simulink model "lineraryzacja"  (R2021b)
settings: Solver=ode45  StartTime=0.0  StopTime=100.0  RelTol=1e-10
values from neighbouring files (symbols this model uses):
  G = 9.81    [edda.m]
  K0 = 1    [edda.m]
  K1 = 1    [edda.m]
  O1 = 3.1    [edda.m]
  O3 = 0.24    [edda.m]
  O4 = 0.77    [edda.m]
settings Model: Creator=mbober  LastModifiedBy=mbober
settings SolverCC: AlgebraicLoopSolver=TrustRegion
settings DebuggingCC: SFMachineParentedDataDiag=warning

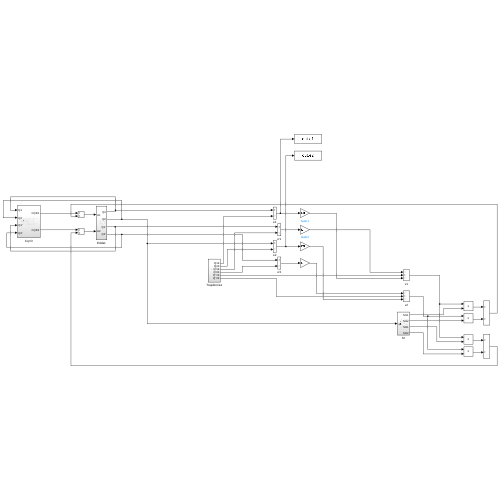
[thumbnail: Simulink's stored preview of the top-level diagram]
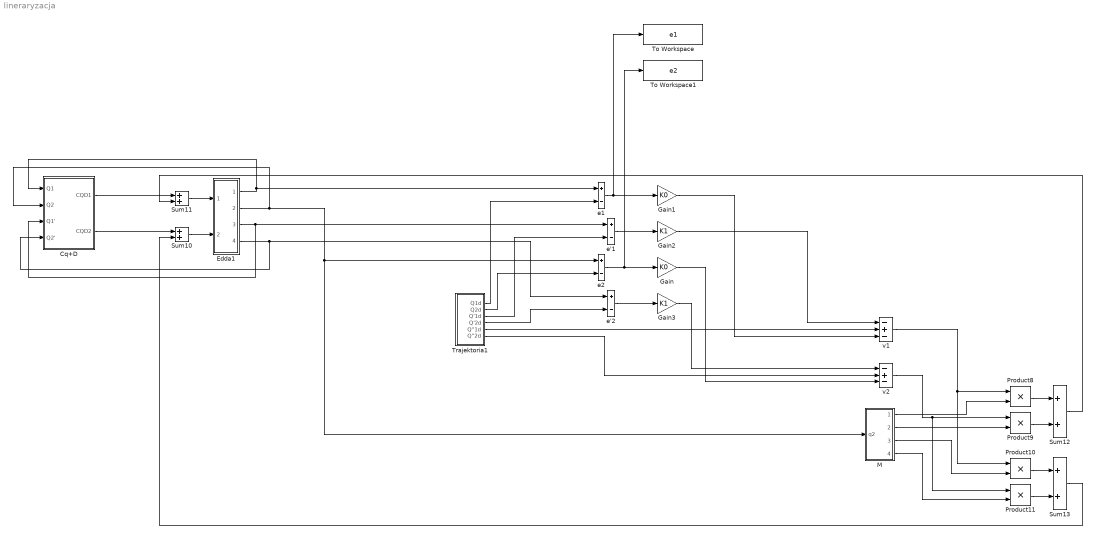
== system lineraryzacja ==
  Cq+D : Subsystem
  Edda1 : Subsystem
  Gain : Gain  Gain=K0
  Gain1 : Gain  Gain=K0
  Gain2 : Gain  Gain=K1
  Gain3 : Gain  Gain=K1
  M : Subsystem
  Product{8..11} (4 alike) : Product
  Sum{10..13} (4 alike) : Sum
  To Workspace : ToWorkspace  VariableName=e1  SampleTime=-1
  To Workspace1 : ToWorkspace  VariableName=e2  SampleTime=-1
  Trajektoria1 : Subsystem
  e'1 : Sum  Inputs=+-
  e'2 : Sum  Inputs=+-
  e1 : Sum  Inputs=+-
  e2 : Sum  Inputs=+-
  v1 : Sum  Inputs=-+-
  v2 : Sum  Inputs=-+-
  wires:
  e1/1 -> Gain1/1, To Workspace/1
  Edda1/1(Q1) -> Cq+D/1(Q1), e1/1
  Edda1/2(Q2) -> Cq+D/2(Q2), e2/1, M/1(q2)
  Sum10/1 -> Edda1/2(U2)
  Sum11/1 -> Edda1/1(U1)
  Trajektoria1/3(Q'1d) -> e'1/2
  Trajektoria1/1(Q1d) -> e1/2
  Trajektoria1/2(Q2d) -> e2/2
  Trajektoria1/4(Q'2d) -> e'2/2
  Trajektoria1/5(Q''1d) -> v1/2
  Trajektoria1/6(Q''2d) -> v2/2
  M/1(M11) -> Product8/2
  v1/1 -> Product10/1, Product8/1
  M/2(M12) -> Product9/2
  v2/1 -> Product11/1, Product9/1
  Product8/1 -> Sum12/1
  Product9/1 -> Sum12/2
  Sum12/1 -> Sum11/2
  Product10/1 -> Sum13/1
  Product11/1 -> Sum13/2
  M/3(M21) -> Product10/2
  M/4(M22) -> Product11/2
  Sum13/1 -> Sum10/2
  Cq+D/1(CQD1) -> Sum11/1
  Cq+D/2(CQD2) -> Sum10/1
  e2/1 -> Gain/1, To Workspace1/1
  Edda1/3(Q1') -> Cq+D/3(Q1'), e'1/1
  Edda1/4(Q2') -> Cq+D/4(Q2'), e'2/1
  Gain1/1 -> v1/3
  Gain/1 -> v2/3
  e'1/1 -> Gain2/1
  e'2/1 -> Gain3/1
  Gain2/1 -> v1/1
  Gain3/1 -> v2/1

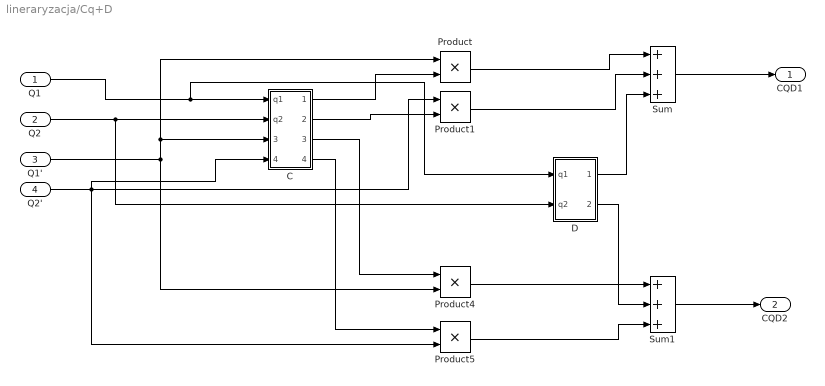
== system lineraryzacja/Cq+D ==
  Q1 : Inport
  Q2 : Inport  Port=2
  Q1' : Inport  Port=3
  Q2' : Inport  Port=4
  C : Subsystem
  D : Subsystem
  Product{,1,4..5} (4 alike) : Product
  Sum : Sum  Inputs=+++
  Sum1 : Sum  Inputs=+++
  CQD1 : Outport
  CQD2 : Outport  Port=2
  wires:
  C/1(C11) -> Product/2
  Q1'/1 -> C/3(q1'), Product/1, Product4/2
  Product/1 -> Sum/1
  Product1/1 -> Sum/2
  C/2(C12) -> Product1/2
  Q2'/1 -> C/4(q2'), Product5/2, Product1/1
  D/1(Out1) -> Sum/3
  C/3(C21) -> Product4/1
  C/4(C22) -> Product5/1
  Product4/1 -> Sum1/1
  Product5/1 -> Sum1/3
  D/2(Out2) -> Sum1/2
  Sum/1 -> CQD1/1
  Sum1/1 -> CQD2/1
  Q1/1 -> D/1(q1), C/1(q1)
  Q2/1 -> D/2(q2), C/2(q2)

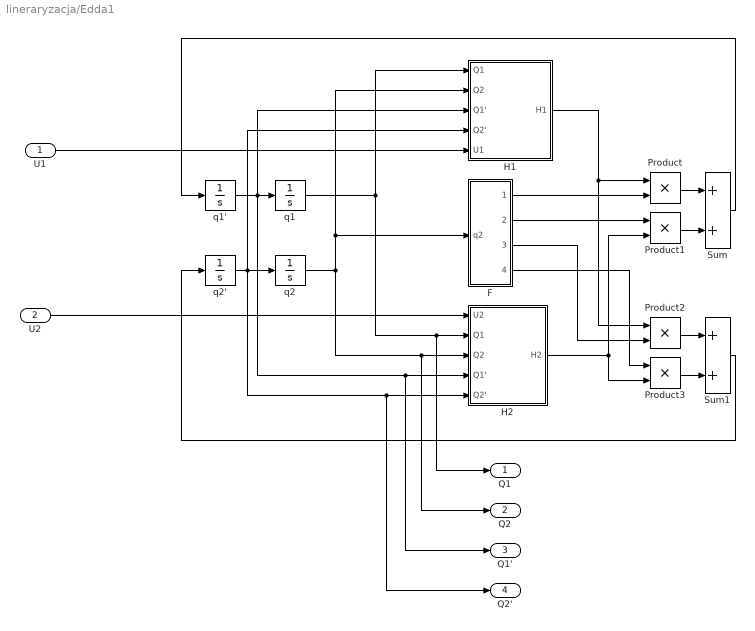
== system lineraryzacja/Edda1 ==
  U1 : Inport
  U2 : Inport  Port=2
  F : Subsystem
  H1 : Subsystem
  H2 : Subsystem
  Product{,1..3} (4 alike) : Product
  Sum : Sum
  Sum1 : Sum
  q1 : Integrator
  q1' : Integrator
  q2 : Integrator
  q2' : Integrator
  Q1 : Outport
  Q2 : Outport  Port=2
  Q1' : Outport  Port=3
  Q2' : Outport  Port=4
  wires:
  Product3/1 -> Sum1/2
  Product/1 -> Sum/1
  q2/1 -> F/1(q2), H1/2(Q2), Q2/1, H2/3(Q2)
  Sum1/1 -> q2'/1
  H1/1(H1) -> Product2/1, Product/1
  q2'/1 -> H1/4(Q2'), Q2'/1, H2/5(Q2'), q2/1
  Sum/1 -> q1'/1
  Product1/1 -> Sum/2
  F/3(F21) -> Product2/2
  H2/1(H2) -> Product3/2, Product1/2
  q1/1 -> H1/1(Q1), Q1/1, H2/2(Q1)
  Product2/1 -> Sum1/1
  F/1(F11) -> Product/2
  U1/1 -> H1/5(U1)
  F/2(F12) -> Product1/1
  q1'/1 -> H1/3(Q1'), Q1'/1, H2/4(Q1'), q1/1
  U2/1 -> H2/1(U2)
  F/4(F22) -> Product3/1

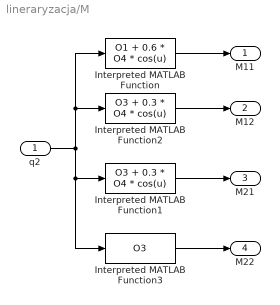
== system lineraryzacja/M ==
  q2 : Inport
  Interpreted MATLAB Function : MATLABFcn  MATLABFcn=O1 + 0.6 * O4 * cos(u)
  Interpreted MATLAB Function1 : MATLABFcn  MATLABFcn=O3 + 0.3 * O4 * cos(u)
  Interpreted MATLAB Function2 : MATLABFcn  MATLABFcn=O3 + 0.3 * O4 * cos(u)
  Interpreted MATLAB Function3 : MATLABFcn  MATLABFcn=O3
  M11 : Outport
  M12 : Outport  Port=2
  M21 : Outport  Port=3
  M22 : Outport  Port=4
  wires:
  Interpreted MATLAB Function3/1 -> M22/1
  Interpreted MATLAB Function/1 -> M11/1
  Interpreted MATLAB Function2/1 -> M12/1
  q2/1 -> Interpreted MATLAB Function/1, Interpreted MATLAB Function2/1, Interpreted MATLAB Function3/1, Interpreted MATLAB Function1/1
  Interpreted MATLAB Function1/1 -> M21/1

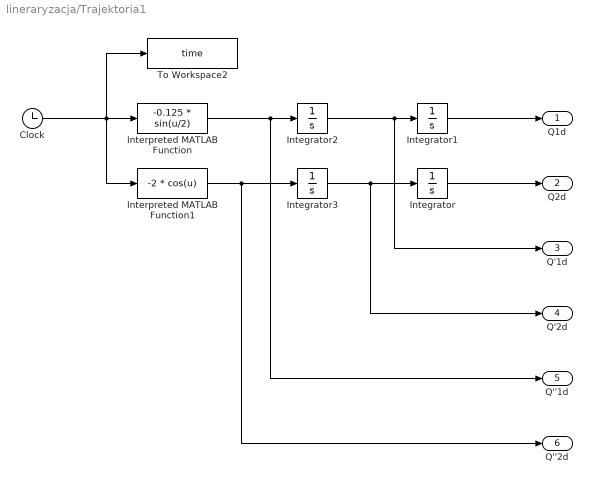
== system lineraryzacja/Trajektoria1 ==
  Clock : Clock
  Integrator : Integrator  InitialCondition=2
  Integrator1 : Integrator
  Integrator2 : Integrator  InitialCondition=0.25
  Integrator3 : Integrator
  Interpreted MATLAB Function : MATLABFcn  MATLABFcn=-0.125 * sin(u/2)
  Interpreted MATLAB Function1 : MATLABFcn  MATLABFcn=-2 * cos(u)
  To Workspace2 : ToWorkspace  VariableName=time  SampleTime=-1
  Q1d : Outport
  Q2d : Outport  Port=2
  Q'1d : Outport  Port=3
  Q'2d : Outport  Port=4
  Q''1d : Outport  Port=5
  Q''2d : Outport  Port=6
  wires:
  Integrator1/1 -> Q1d/1
  Interpreted MATLAB Function/1 -> Q''1d/1, Integrator2/1
  Integrator/1 -> Q2d/1
  Interpreted MATLAB Function1/1 -> Q''2d/1, Integrator3/1
  Clock/1 -> To Workspace2/1, Interpreted MATLAB Function1/1, Interpreted MATLAB Function/1
  Integrator2/1 -> Q'1d/1, Integrator1/1
  Integrator3/1 -> Q'2d/1, Integrator/1

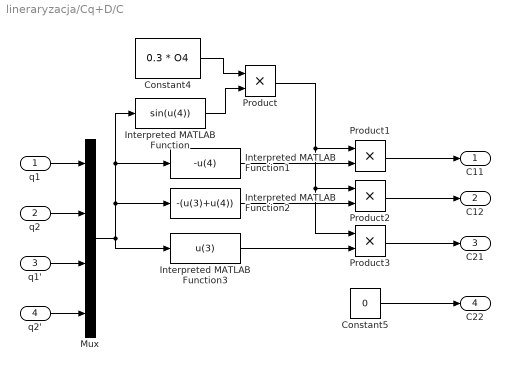
== system lineraryzacja/Cq+D/C ==
  q1 : Inport
  q2 : Inport  Port=2
  q1' : Inport  Port=3
  q2' : Inport  Port=4
  Constant4 : Constant  Value=0.3 * O4
  Constant5 : Constant  Value=0
  Interpreted MATLAB Function : MATLABFcn  MATLABFcn=sin(u(4))
  Interpreted MATLAB Function1 : MATLABFcn  MATLABFcn=-u(4)
  Interpreted MATLAB Function2 : MATLABFcn  MATLABFcn=-(u(3)+u(4))
  Interpreted MATLAB Function3 : MATLABFcn  MATLABFcn=u(3)
  Mux : Mux
  Product{,1..3} (4 alike) : Product
  C11 : Outport
  C12 : Outport  Port=2
  C21 : Outport  Port=3
  C22 : Outport  Port=4
  wires:
  Product3/1 -> C21/1
  Interpreted MATLAB Function1/1 -> Product1/2
  q2'/1 -> Mux/4
  Interpreted MATLAB Function2/1 -> Product2/2
  q2/1 -> Mux/2
  Constant4/1 -> Product/1
  Interpreted MATLAB Function/1 -> Product/2
  Product1/1 -> C11/1
  Interpreted MATLAB Function3/1 -> Product3/2
  q1'/1 -> Mux/3
  Mux/1 -> Interpreted MATLAB Function3/1, Interpreted MATLAB Function2/1, Interpreted MATLAB Function/1, Interpreted MATLAB Function1/1
  q1/1 -> Mux/1
  Constant5/1 -> C22/1
  Product/1 -> Product3/1, Product2/1, Product1/1
  Product2/1 -> C12/1

== system lineraryzacja/Cq+D/D ==
  q1 : Inport
  q2 : Inport  Port=2
  Interpreted MATLAB Function : MATLABFcn  MATLABFcn=(O1 * cos(u(2)) + O4 * cos(u(1)*u(2))) * G
  Interpreted MATLAB Function1 : MATLABFcn  MATLABFcn=O4 * cos(u(1)*u(2)) * G
  Mux : Mux  Inputs=2
  Out1 : Outport
  Out2 : Outport  Port=2
  wires:
  Interpreted MATLAB Function/1 -> Out1/1
  Interpreted MATLAB Function1/1 -> Out2/1
  Mux/1 -> Interpreted MATLAB Function1/1, Interpreted MATLAB Function/1
  q1/1 -> Mux/1
  q2/1 -> Mux/2

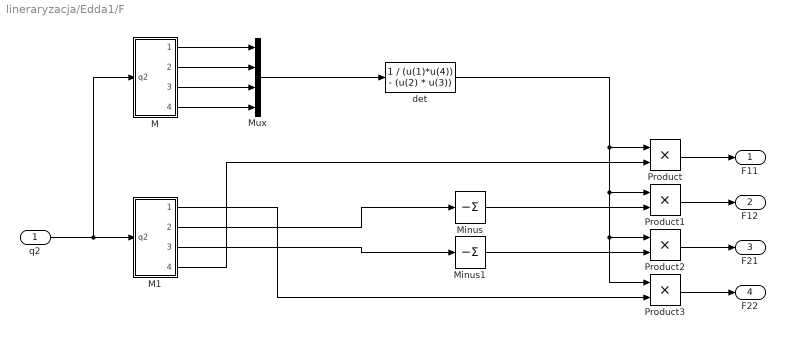
== system lineraryzacja/Edda1/F ==
  q2 : Inport
  M : Subsystem
  M1 : Subsystem
  Minus : Sum  Inputs=-
  Minus1 : Sum  Inputs=-
  Mux : Mux
  Product{,1..3} (4 alike) : Product
  det : MATLABFcn  MATLABFcn=1 / (u(1)*u(4)) - (u(2) * u(3))
  F11 : Outport
  F12 : Outport  Port=2
  F21 : Outport  Port=3
  F22 : Outport  Port=4
  wires:
  q2/1 -> M/1(q2), M1/1(q2)
  M1/2(M12) -> Minus/1
  M1/3(M21) -> Minus1/1
  Mux/1 -> det/1
  M/2(M12) -> Mux/2
  M/1(M11) -> Mux/1
  M/3(M21) -> Mux/3
  M/4(M22) -> Mux/4
  Product/1 -> F11/1
  Product1/1 -> F12/1
  Product2/1 -> F21/1
  Product3/1 -> F22/1
  det/1 -> Product3/1, Product2/1, Product1/1, Product/1
  M1/1(M11) -> Product3/2
  M1/4(M22) -> Product/2
  Minus/1 -> Product1/2
  Minus1/1 -> Product2/2

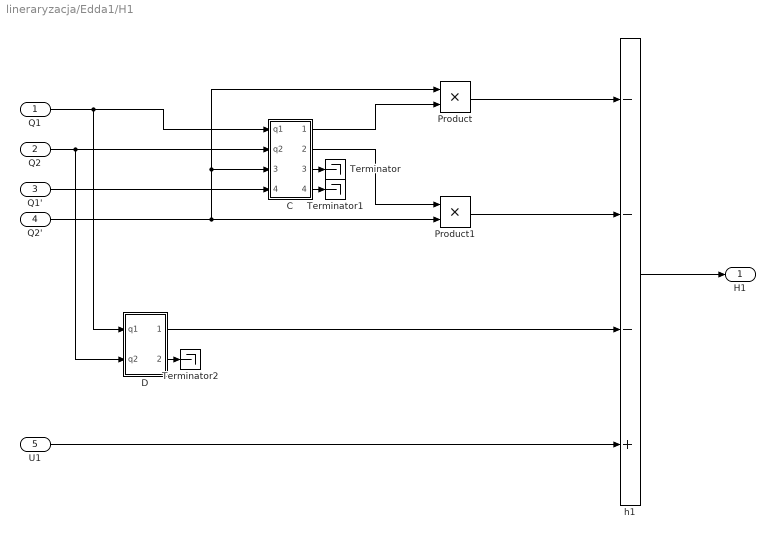
== system lineraryzacja/Edda1/H1 ==
  Q1 : Inport
  Q2 : Inport  Port=2
  Q1' : Inport  Port=3
  Q2' : Inport  Port=4
  U1 : Inport  Port=5
  C : Subsystem
  D : Subsystem
  Product : Product
  Product1 : Product
  Terminator : Terminator
  Terminator1 : Terminator
  Terminator2 : Terminator
  h1 : Sum  Inputs=---+
  H1 : Outport
  wires:
  U1/1 -> h1/4
  C/2(C12) -> Product1/1
  Product/1 -> h1/1
  Q1'/1 -> C/3(q1'), Product/1
  Product1/1 -> h1/2
  Q2/1 -> D/2(q2), C/2(q2)
  C/1(C11) -> Product/2
  Q1/1 -> D/1(q1), C/1(q1)
  D/1(Out1) -> h1/3
  Q2'/1 -> C/4(q2'), Product1/2
  h1/1 -> H1/1
  C/3(C21) -> Terminator/1
  C/4(C22) -> Terminator1/1
  D/2(Out2) -> Terminator2/1

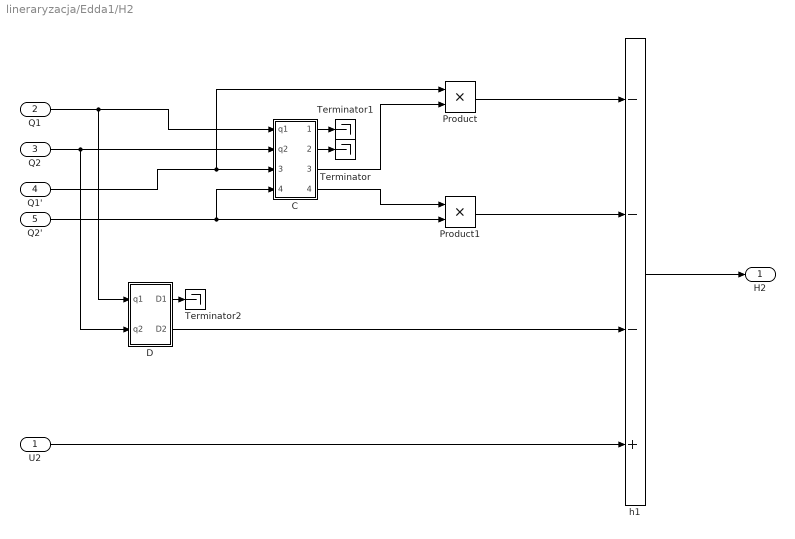
== system lineraryzacja/Edda1/H2 ==
  U2 : Inport
  Q1 : Inport  Port=2
  Q2 : Inport  Port=3
  Q1' : Inport  Port=4
  Q2' : Inport  Port=5
  C : Subsystem
  D : Subsystem
  Product : Product
  Product1 : Product
  Terminator : Terminator
  Terminator1 : Terminator
  Terminator2 : Terminator
  h1 : Sum  Inputs=---+
  H2 : Outport
  wires:
  C/3(C21) -> Product/2
  U2/1 -> h1/4
  C/4(C22) -> Product1/1
  Product1/1 -> h1/2
  D/2(D2) -> h1/3
  Product/1 -> h1/1
  Q2/1 -> D/2(q2), C/2(q2)
  Q2'/1 -> C/4(q2'), Product1/2
  h1/1 -> H2/1
  Q1'/1 -> C/3(q1'), Product/1
  Q1/1 -> D/1(q1), C/1(q1)
  C/2(C12) -> Terminator/1
  C/1(C11) -> Terminator1/1
  D/1(D1) -> Terminator2/1

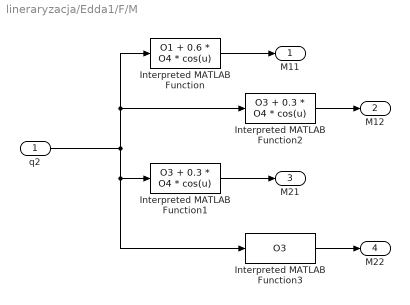
== system lineraryzacja/Edda1/F/M ==
  q2 : Inport
  Interpreted MATLAB Function : MATLABFcn  MATLABFcn=O1 + 0.6 * O4 * cos(u)
  Interpreted MATLAB Function1 : MATLABFcn  MATLABFcn=O3 + 0.3 * O4 * cos(u)
  Interpreted MATLAB Function2 : MATLABFcn  MATLABFcn=O3 + 0.3 * O4 * cos(u)
  Interpreted MATLAB Function3 : MATLABFcn  MATLABFcn=O3
  M11 : Outport
  M12 : Outport  Port=2
  M21 : Outport  Port=3
  M22 : Outport  Port=4
  wires:
  Interpreted MATLAB Function3/1 -> M22/1
  Interpreted MATLAB Function/1 -> M11/1
  Interpreted MATLAB Function2/1 -> M12/1
  q2/1 -> Interpreted MATLAB Function/1, Interpreted MATLAB Function2/1, Interpreted MATLAB Function3/1, Interpreted MATLAB Function1/1
  Interpreted MATLAB Function1/1 -> M21/1

== system lineraryzacja/Edda1/F/M1 ==
  q2 : Inport
  Interpreted MATLAB Function : MATLABFcn  MATLABFcn=O1 + 0.6 * O4 * cos(u)
  Interpreted MATLAB Function1 : MATLABFcn  MATLABFcn=O3 + 0.3 * O4 * cos(u)
  Interpreted MATLAB Function2 : MATLABFcn  MATLABFcn=O3 + 0.3 * O4 * cos(u)
  Interpreted MATLAB Function3 : MATLABFcn  MATLABFcn=O3
  M11 : Outport
  M12 : Outport  Port=2
  M21 : Outport  Port=3
  M22 : Outport  Port=4
  wires:
  Interpreted MATLAB Function3/1 -> M22/1
  Interpreted MATLAB Function/1 -> M11/1
  Interpreted MATLAB Function2/1 -> M12/1
  q2/1 -> Interpreted MATLAB Function/1, Interpreted MATLAB Function2/1, Interpreted MATLAB Function3/1, Interpreted MATLAB Function1/1
  Interpreted MATLAB Function1/1 -> M21/1

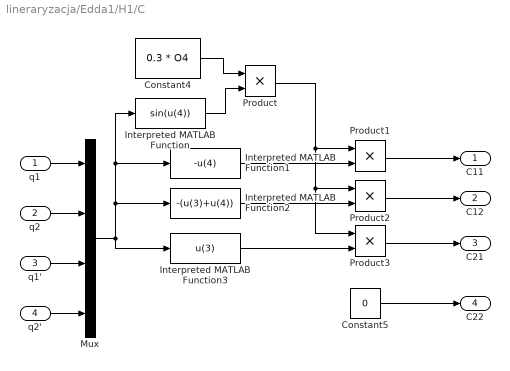
== system lineraryzacja/Edda1/H1/C ==
  q1 : Inport
  q2 : Inport  Port=2
  q1' : Inport  Port=3
  q2' : Inport  Port=4
  Constant4 : Constant  Value=0.3 * O4
  Constant5 : Constant  Value=0
  Interpreted MATLAB Function : MATLABFcn  MATLABFcn=sin(u(4))
  Interpreted MATLAB Function1 : MATLABFcn  MATLABFcn=-u(4)
  Interpreted MATLAB Function2 : MATLABFcn  MATLABFcn=-(u(3)+u(4))
  Interpreted MATLAB Function3 : MATLABFcn  MATLABFcn=u(3)
  Mux : Mux
  Product{,1..3} (4 alike) : Product
  C11 : Outport
  C12 : Outport  Port=2
  C21 : Outport  Port=3
  C22 : Outport  Port=4
  wires:
  Product3/1 -> C21/1
  Interpreted MATLAB Function1/1 -> Product1/2
  q2'/1 -> Mux/4
  Interpreted MATLAB Function2/1 -> Product2/2
  q2/1 -> Mux/2
  Constant4/1 -> Product/1
  Interpreted MATLAB Function/1 -> Product/2
  Product1/1 -> C11/1
  Interpreted MATLAB Function3/1 -> Product3/2
  q1'/1 -> Mux/3
  Mux/1 -> Interpreted MATLAB Function3/1, Interpreted MATLAB Function2/1, Interpreted MATLAB Function/1, Interpreted MATLAB Function1/1
  q1/1 -> Mux/1
  Constant5/1 -> C22/1
  Product/1 -> Product3/1, Product2/1, Product1/1
  Product2/1 -> C12/1

== system lineraryzacja/Edda1/H1/D ==
  q1 : Inport
  q2 : Inport  Port=2
  Interpreted MATLAB Function : MATLABFcn  MATLABFcn=(O1 * cos(u(2)) + O4 * cos(u(1)*u(2))) * G
  Interpreted MATLAB Function1 : MATLABFcn  MATLABFcn=O4 * cos(u(1)*u(2)) * G
  Mux : Mux  Inputs=2
  Out1 : Outport
  Out2 : Outport  Port=2
  wires:
  Interpreted MATLAB Function/1 -> Out1/1
  Interpreted MATLAB Function1/1 -> Out2/1
  Mux/1 -> Interpreted MATLAB Function1/1, Interpreted MATLAB Function/1
  q1/1 -> Mux/1
  q2/1 -> Mux/2

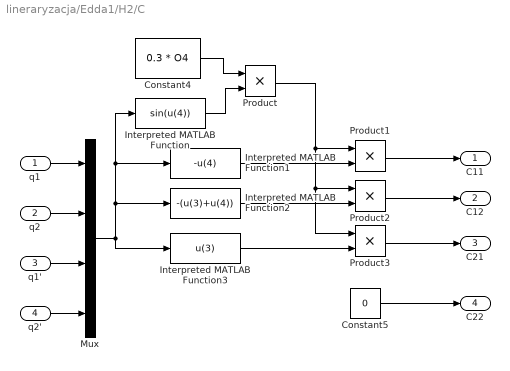
== system lineraryzacja/Edda1/H2/C ==
  q1 : Inport
  q2 : Inport  Port=2
  q1' : Inport  Port=3
  q2' : Inport  Port=4
  Constant4 : Constant  Value=0.3 * O4
  Constant5 : Constant  Value=0
  Interpreted MATLAB Function : MATLABFcn  MATLABFcn=sin(u(4))
  Interpreted MATLAB Function1 : MATLABFcn  MATLABFcn=-u(4)
  Interpreted MATLAB Function2 : MATLABFcn  MATLABFcn=-(u(3)+u(4))
  Interpreted MATLAB Function3 : MATLABFcn  MATLABFcn=u(3)
  Mux : Mux
  Product{,1..3} (4 alike) : Product
  C11 : Outport
  C12 : Outport  Port=2
  C21 : Outport  Port=3
  C22 : Outport  Port=4
  wires:
  Product3/1 -> C21/1
  Interpreted MATLAB Function1/1 -> Product1/2
  q2'/1 -> Mux/4
  Interpreted MATLAB Function2/1 -> Product2/2
  q2/1 -> Mux/2
  Constant4/1 -> Product/1
  Interpreted MATLAB Function/1 -> Product/2
  Product1/1 -> C11/1
  Interpreted MATLAB Function3/1 -> Product3/2
  q1'/1 -> Mux/3
  Mux/1 -> Interpreted MATLAB Function3/1, Interpreted MATLAB Function2/1, Interpreted MATLAB Function/1, Interpreted MATLAB Function1/1
  q1/1 -> Mux/1
  Constant5/1 -> C22/1
  Product/1 -> Product3/1, Product2/1, Product1/1
  Product2/1 -> C12/1

== system lineraryzacja/Edda1/H2/D ==
  q1 : Inport
  q2 : Inport  Port=2
  Interpreted MATLAB Function : MATLABFcn  MATLABFcn=(O1 * cos(u(2)) + O4 * cos(u(1)*u(2))) * G
  Interpreted MATLAB Function1 : MATLABFcn  MATLABFcn=O4 * cos(u(1)*u(2)) * G
  Mux : Mux  Inputs=2
  D1 : Outport
  D2 : Outport  Port=2
  wires:
  Interpreted MATLAB Function/1 -> D1/1
  Interpreted MATLAB Function1/1 -> D2/1
  Mux/1 -> Interpreted MATLAB Function1/1, Interpreted MATLAB Function/1
  q1/1 -> Mux/1
  q2/1 -> Mux/2
